simulink model "modelo_convergencia_balance_1gdl"  (R2022b)
settings: Solver=VariableStepAuto  StartTime=0.0  StopTime=20  RelTol=1e-3
values from neighbouring files (symbols this model uses):
  G_act = tf([1],[tauc+taum,1])    [SAS.m]
  K_DL = 1/FT_conv_balance_1gdl.Kstatic    [SAS.m]
  p = polyfit(time,y,20)    [rise_delay.m]
settings Model: Creator=abelu  LastModifiedBy=abelu

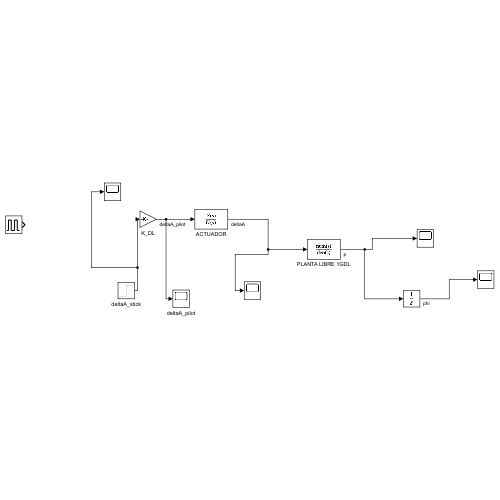
[thumbnail: Simulink's stored preview of the top-level diagram]
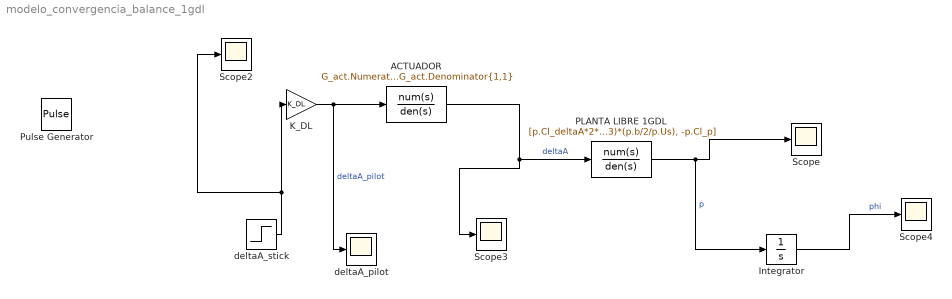
== system modelo_convergencia_balance_1gdl ==
  ACTUADOR : TransferFcn  Numerator=G_act.Numerator{1,1}  Denominator=G_act.Denominator{1,1}
  Integrator : Integrator
  K_DL : Gain  Gain=K_DL
  PLANTA LIBRE 1GDL : TransferFcn  Numerator=[p.Cl_deltaA*2*p.Us/p.b]  Denominator=[p.I_xx/(p.rhos*p.Sw*(p.b/2)^3)*(p.b/2/p.Us), -p.Cl_p]
  Pulse Generator : DiscretePulseGenerator  PulseType=Time based  Period=200  PulseWidth=5
  Scope{,2..4} (4 alike) : Scope
  deltaA_pilot : Scope
  deltaA_stick : Step  Time=0  SampleTime=0
  wires:
  PLANTA LIBRE 1GDL/1 -> Integrator/1, Scope/1  "p"
  deltaA_stick/1 -> Scope2/1, K_DL/1
  K_DL/1 -> deltaA_pilot/1, ACTUADOR/1  "deltaA_pilot"
  ACTUADOR/1 -> Scope3/1, PLANTA LIBRE 1GDL/1  "deltaA"
  Integrator/1 -> Scope4/1  "phi"
